simulink model "nine_g"  (R2025a)
settings: Solver=FixedStepDiscrete  StartTime=0.0  StopTime=1  FixedStep=1  RelTol=1e-3
model workspace (MAT data in the model file):
  y = -1
settings Model: Creator=horty  LastModifiedBy=sdarshan
settings DataIOCC: SaveFormat=Array  SignalLogging=off  DSMLogging=off  SaveTime=off  ReturnWorkspaceOutputs=off

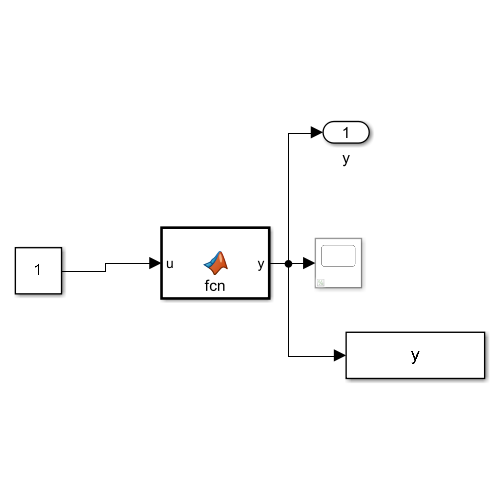
[thumbnail: Simulink's stored preview of the top-level diagram]
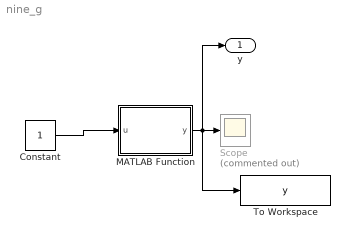
== system nine_g ==
  Constant : Constant
  MATLAB Function : MATLAB Function  TreatAsAtomicUnit=on
  Scope : Scope  Commented=on
      settings: ActiveDisplayYMinimum=0.9  ActiveDisplayYMaximum=1.1
  To Workspace : ToWorkspace  VariableName=y  SampleTime=-1
      settings: MaxDataPoints=1  Save2DSignal=2-D array (concatenate along first dimension)
  y : Outport
  wires:
  Constant/1 -> MATLAB Function/1(u)
  MATLAB Function/1(y) -> y/1, To Workspace/1, Scope/1

== matlab function nine_g/MATLAB Function ==
  data: u input; y output
function y = fcn(u)
%Implement structural analysis code to test if wingbox can sustain 9g
%loads. 
y = u;
